simulink model "H7_new_series_switching_upcoming_conference"  (R2018a)
settings: Solver=ode45  StartTime=0.0  StopTime=2  RelTol=1e-3  EnableMultiTasking=on
libraries: powerlib x23, powerlib_extras x3, powerlib_meascontrol x3, simulink x1
settings Model: Creator=Personal  LastModifiedBy=HP
settings DataIOCC: LimitDataPoints=on  SaveFormat=Array
settings OptimizationCC: LifeSpan=inf
settings DebuggingCC: SolverPrmCheckMsg=warning  SFUnexpectedBacktrackingDiag=warning  SFNoUnconditionalDefaultTransitionDiag=warning  SFExecutionAtInitializationDiag=none
settings HardwareCC: ProdBitPerPointer=32  ProdBitPerSizeT=32  ProdBitPerPtrDiffT=32  ProdLargestAtomicFloat=None  ProdIntDivRoundTo=Undefined  ProdEndianess=Unspecified  ProdWordSize=32  ProdHWDeviceType=32-bit Generic
settings ModelReferenceCC: PropagateSignalLabelsOutOfModel=off
settings CodeAppCC: StateflowObjectComments=on
settings GRTTargetCC: TargetLangStandard=C89/C90 (ANSI)  GeneratePreprocessorConditionals=Disable all
settings ConfigComp: CovMetricSettings=dw  CovHtmlReporting=on  CovSaveCumulativeToWorkspaceVar=on  CovSaveSingleToWorkspaceVar=on  CovExternalEMLEnable=off  CovSFcnEnable=off
settings SimscapeCC: SimscapeNormalizeSystem=off

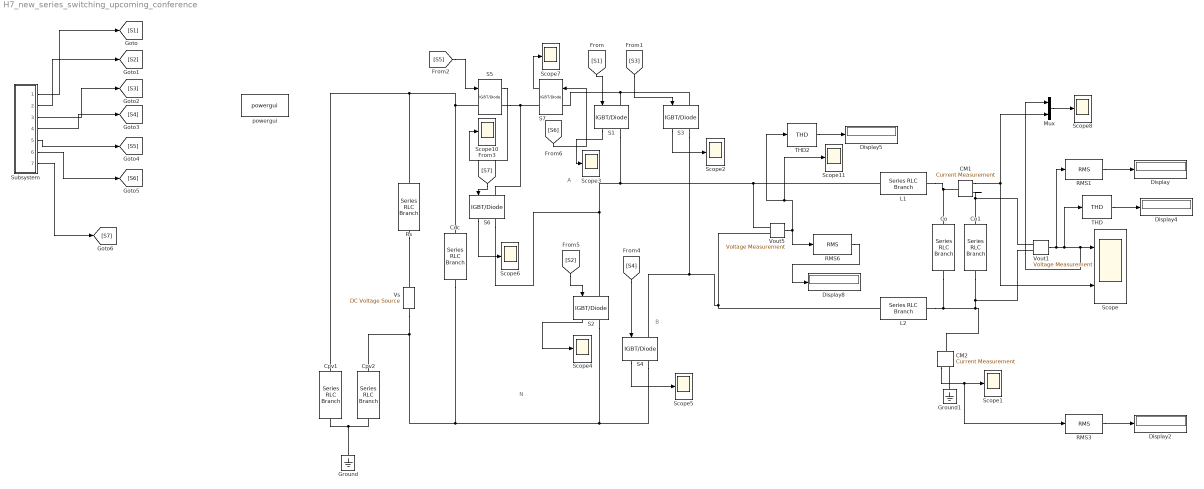
== system H7_new_series_switching_upcoming_conference ==
  note: A
  note: N
  note: B
  CM1 : powerlib/Measurements/Current Measurement  PhasorSimulation=off  OutputType=Complex  PSBequivalent=0
  CM2 : powerlib/Measurements/Current Measurement  PhasorSimulation=off  OutputType=Complex  PSBequivalent=0
  Cdc : powerlib/Elements/Series RLC Branch  LConnTagsString=__new0  RConnTagsString=__new0  BranchType=C  Resistance=1  Inductance=3e-3  SetiL0=off  InitialCurrent=0  Capacitance=940e-6  Setx0=off  InitialVoltage=0  Measurements=None
  Co : powerlib/Elements/Series RLC Branch  LConnTagsString=__new0  RConnTagsString=__new0  BranchType=C  Resistance=1  Inductance=3e-3  SetiL0=off  InitialCurrent=0  Capacitance=2.2e-6  Setx0=off  InitialVoltage=0  Measurements=None
  Co1 : powerlib/Elements/Series RLC Branch  LConnTagsString=__new0  RConnTagsString=__new0  BranchType=R  Resistance=5  Inductance=3e-3  SetiL0=off  InitialCurrent=0  Capacitance=2.2e-6  Setx0=off  InitialVoltage=0  Measurements=None
  Cpv1 : powerlib/Elements/Series RLC Branch  LConnTagsString=__new0  RConnTagsString=__new0  BranchType=C  Resistance=1  Inductance=3e-3  SetiL0=off  InitialCurrent=0  Capacitance=75e-9  Setx0=off  InitialVoltage=0  Measurements=None
  Cpv2 : powerlib/Elements/Series RLC Branch  LConnTagsString=__new0  RConnTagsString=__new0  BranchType=C  Resistance=1  Inductance=3e-3  SetiL0=off  InitialCurrent=0  Capacitance=75e-9  Setx0=off  InitialVoltage=0  Measurements=None
  Display{,2,4..5,8} (5 alike) : Display
  Ground : powerlib/Elements/Ground  LConnTagsString=a
  Ground1 : powerlib/Elements/Ground  LConnTagsString=a
  L1 : powerlib/Elements/Series RLC Branch  LConnTagsString=__new0  RConnTagsString=__new0  BranchType=L  Resistance=1  Inductance=3e-3  SetiL0=off  InitialCurrent=0  Capacitance=1e-6  Setx0=off  InitialVoltage=0  Measurements=None
  L2 : powerlib/Elements/Series RLC Branch  LConnTagsString=__new0  RConnTagsString=__new0  BranchType=L  Resistance=1  Inductance=3e-3  SetiL0=off  InitialCurrent=0  Capacitance=1e-6  Setx0=off  InitialVoltage=0  Measurements=None
  Mux : Mux  Inputs=2
  RMS1 : powerlib_extras/Measurements/RMS  f1=50
  RMS3 : powerlib_extras/Measurements/RMS  f1=50
  RMS6 : powerlib_extras/Measurements/RMS  f1=50
  Rs : powerlib/Elements/Series RLC Branch  LConnTagsString=__new0  RConnTagsString=__new0  BranchType=R  Resistance=1  Inductance=3e-3  SetiL0=off  InitialCurrent=0  Capacitance=1e-6  Setx0=off  InitialVoltage=0  Measurements=None
  S{1..7} (7 alike) : powerlib/Power Electronics/IGBT//Diode  Ron=1e-3  Rs=1e5  Cs=inf  Measurements=on
  Scope : Scope  NumInputPorts=2
  Scope{1..8,10..11} (10 alike) : Scope
  Subsystem : Subsystem
  THD : powerlib_meascontrol/Measurements/THD  Freq=50  Ts=0
  THD2 : powerlib_meascontrol/Measurements/THD  Freq=60  Ts=0
  Vout1 : powerlib/Measurements/Voltage Measurement  PhasorSimulation=off  OutputType=Complex  PSBequivalent=0
  Vout5 : powerlib/Measurements/Voltage Measurement  PhasorSimulation=off  OutputType=Complex  PSBequivalent=0
  Vs : powerlib/Electrical Sources/DC Voltage Source  Amplitude=330  Measurements=None
  powergui : powerlib/powergui  Priority=1  SimulationMode=Continuous  SampleTime=50e-6  frequency=60  Iterations=50  frequencyindice=0  Pbase=100e6  ErrMax=1e-4  UnitsV=kV  UnitsW=MW  buscounter=0  FunctionMessages=off  echomessages=off  EnableUseOfTLC=off  CurrentSourceSwitches=off  DisableSnubberDevices=off  DisableRonSwitches=off  DisableVfSwitches=off  DisplayEquations=off  SolverType=Tustin/Backward Euler (TBE)  Interpol=off  ExternalGateDelay=off  methode=off  Ts=100  x0status=blocks  SPID=on  SwTol=0  HookPort=off  RestoreLinks=warning  ResistiveCurrentMeasurement=off  Frange=[0:2:500]  Ylog=off  Xlog=on  ShowGrid=off  save=off  variable=ZData  structure=THD  ZoomFFT=off  StartTime=1  cycles=5  DisplayStyle=1  fundamental=50  FreqAxis=off  MaxFrequency=10000  frequencyindicesteady=1  RmsSteady=1  display=off
  wires:
  Subsystem/1(Out1) -> [S1]
  Subsystem/2(Out2) -> [S2]
  Subsystem/3(Out3) -> [S3]
  Subsystem/4(Out4) -> [S4]
  Subsystem/5(Out5) -> [S5]
  [S1] -> S1/1
  [S3] -> S3/1
  Vout1/1 -> RMS1/1, THD/1, Mux/1, Scope/1
  THD/1 -> Display4/1
  [S4] -> S4/1
  [S2] -> S2/1
  RMS3/1 -> Display2/1
  CM2/1 -> RMS3/1, Scope1/1
  RMS1/1 -> Display/1
  THD2/1 -> Display5/1
  Vout5/1 -> Scope11/1, THD2/1, RMS6/1
  RMS6/1 -> Display8/1
  CM1/1 -> Mux/2, Scope/2
  S3/1 -> Scope2/1
  S1/1 -> Scope3/1
  S2/1 -> Scope4/1
  S4/1 -> Scope5/1
  S5/1 -> Scope10/1
  [S5] -> S5/1
  S6/1 -> Scope6/1
  [S7] -> S6/1
  S7/1 -> Scope7/1
  [S6] -> S7/1
  Subsystem/6(Out6) -> [S6]
  Subsystem/7(Out7) -> [S7]
  Mux/1 -> Scope8/1
  connections:
  Cdc/LConn1 -- Rs/RConn1 -- Cpv1/LConn1 -- S5/LConn1
  S1/RConn1 -- S6/RConn1 -- S2/LConn1 -- Vout5/LConn1 -- L1/LConn1
  Ground/LConn1 -- Cpv2/RConn1 -- Cpv1/RConn1
  Vout5/LConn2 -- L2/LConn1 -- S4/LConn1 -- S3/RConn1
  Ground1/LConn1 -- CM2/RConn1
  Rs/LConn1 -- Vs/RConn1
  Vs/LConn1 -- S4/RConn1 -- S2/RConn1 -- Cdc/RConn1 -- Cpv2/LConn1
  L1/RConn1 -- CM1/LConn1 -- Co/LConn1
  L2/RConn1 -- Co/RConn1 -- Co1/RConn1 -- Vout1/LConn2 -- CM2/LConn1
  CM1/RConn1 -- Co1/LConn1 -- Vout1/LConn1
  S5/RConn1 -- S7/RConn1 -- S6/LConn1
  S3/LConn1 -- S1/LConn1 -- S7/LConn1

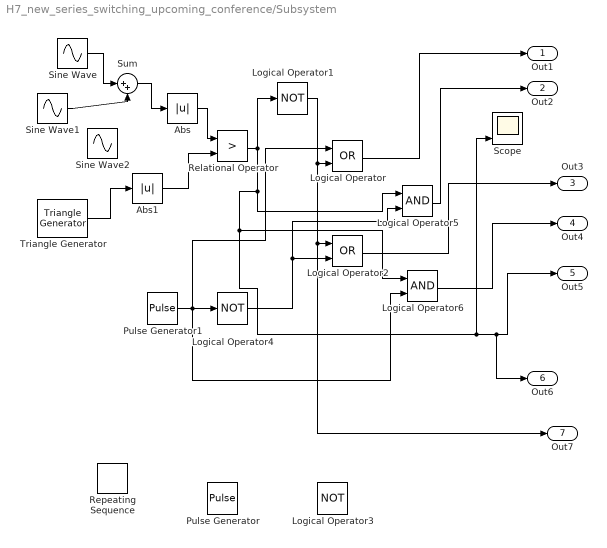
== system H7_new_series_switching_upcoming_conference/Subsystem ==
  Abs : Abs
  Abs1 : Abs
  Logical Operator : Logic  Operator=OR  AllPortsSameDT=off  OutDataTypeStr=boolean
  Logical Operator1 : Logic  Operator=NOT  AllPortsSameDT=off  OutDataTypeStr=boolean
  Logical Operator2 : Logic  Operator=OR  AllPortsSameDT=off  OutDataTypeStr=boolean
  Logical Operator3 : Logic  Operator=NOT  AllPortsSameDT=off  OutDataTypeStr=boolean
  Logical Operator4 : Logic  Operator=NOT  AllPortsSameDT=off  OutDataTypeStr=boolean
  Logical Operator5 : Logic  AllPortsSameDT=off  OutDataTypeStr=boolean
  Logical Operator6 : Logic  AllPortsSameDT=off  OutDataTypeStr=boolean
  Pulse Generator : DiscretePulseGenerator  PulseType=Time based  Period=.02  PulseWidth=50
  Pulse Generator1 : DiscretePulseGenerator  PulseType=Time based  Period=.02  PulseWidth=50
  Relational Operator : RelationalOperator  Operator=>  OutDataTypeStr=boolean  RndMeth=Nearest
  Repeating Sequence : simulink/Sources/Repeating Sequence  rep_seq_t=[0 1]*(1/20000)  rep_seq_y=[0 1]
  Scope : Scope  NumInputPorts=3
  Sine Wave : Sin  Frequency=2*pi*50  SampleTime=0
  Sine Wave1 : Sin  Amplitude=.003  Frequency=2*pi*3*50  Phase=pi  SampleTime=0
  Sine Wave2 : Sin  Amplitude=.001  Frequency=2*pi*5*50  Phase=pi  SampleTime=0
  Sum : Sum  Inputs=|++
  Triangle Generator : powerlib_meascontrol/Pulse & Signal Generators/Triangle Generator  Freq=8e3  Phase=90  Ts=0
  Out1 : Outport
  Out2 : Outport  Port=2
  Out3 : Outport  Port=3
  Out4 : Outport  Port=4
  Out5 : Outport  Port=5
  Out6 : Outport  Port=6
  Out7 : Outport  Port=7
  wires:
  Triangle Generator/1 -> Abs1/1
  Relational Operator/1 -> Logical Operator5/1, Logical Operator6/1, Out6/1, Out5/1, Scope/3, Logical Operator1/1
  Abs1/1 -> Relational Operator/2
  Abs/1 -> Relational Operator/1
  Sine Wave/1 -> Sum/1
  Sine Wave1/1 -> Sum/2
  Sum/1 -> Abs/1
  Pulse Generator1/1 -> Logical Operator/1, Logical Operator6/2, Logical Operator4/1
  Logical Operator4/1 -> Logical Operator5/2, Logical Operator2/2
  Logical Operator1/1 -> Logical Operator/2, Out7/1, Logical Operator2/1
  Logical Operator/1 -> Out1/1
  Logical Operator2/1 -> Out3/1
  Logical Operator6/1 -> Out4/1
  Logical Operator5/1 -> Out2/1
